simulink library "fordypningsprosjekt"  (Simulink 7.1)
values from neighbouring files (symbols this model uses):
  noise = variance.*randn(6,1)    [camsim3.m]
undefined symbols (not defined in the file or in its folder): bottom_signature, C_calc, ekf2, kalmanfilter, kalmanfilter2
libraries: marine_gnc x5, simulink_extras x3, vrlib x2, simulink x1
(part 1 of 2)
settings Model: Creator=anderga  LastModifiedBy=anderga

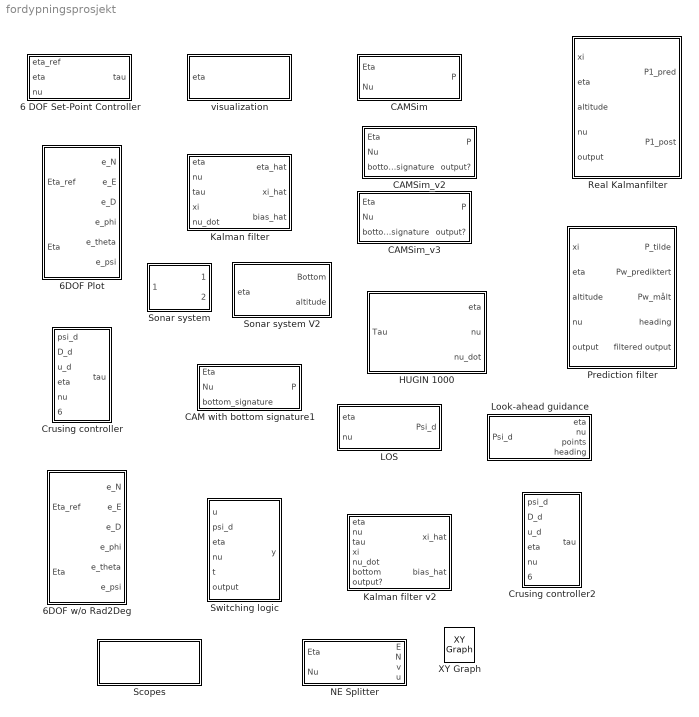
== system fordypningsprosjekt ==
  6 DOF Set-Point Controller : Subsystem  mask(6 DOF Set-point controller){Kp=diag([230 300 1000]), Ki=diag([2 5 0]), Kd=diag([750 700 0]), depthPID=[50, 1, 0], rollPID=[0, 0, 0], pitchPID=[500, 2, 50], sat=1000.*[1, 1, 1, 1, 1, 1]}
      mask prompts: Kp "NE-yaw PID Kp"; Ki "NE-yaw PID Ki"; Kd "NE-yaw PID Kd"; depthPID "Depth PID ([Kp, Ki, Kd])"; rollPID "Roll PID ([Kp, Ki, Kd]) Usually zero, no control moments in roll"; pitchPID "Pitch PID ([Kp, Ki, Kd])"; sat "Forces and Moments Saturation[X, Y, Z, K, M, N]"
      mask init:
      | if isempty(Kp)
      |     Kp = diag([230 300 1000]);
      | end
      | if isempty(Kd)
      |     Kd = diag([750 700 0]);
      | end
      | if isempty(Ki)
      |     Ki = diag([2 5 0]);
      | end
      | if isempty(depthPID)
      |     depthPID = [50, 1, 0];
      | end
      | if isempty(rollPID)
      |     rollPID = [0 0 0];
      | end
      | if isempty(pitchPID)
      |     pitchPID = [500, 2, 50];
      | end
  6DOF Plot : Subsystem
      mask Type: 6 DOF plot reference versus eta
  6DOF w/o Rad2Deg : Subsystem  AncestorBlock=fordypningsprosjekt/6DOF Plot
      mask Type: 6 DOF plot reference versus eta
  CAM with bottom signature1 : Subsystem  AncestorBlock=fordypningsprosjekt/CAM with bottom signature  mask(CAMSim){Noise=off, Variance=0}
      mask prompts: Noise "Noise?"; Variance "Variance noise"
      mask help: Outputs 3 points along the pipeline in the field of view
  CAMSim : Subsystem  mask(CAMSim){bottom=10}
      mask prompts: bottom "Sea Bottom [m]"
      mask help: Outputs 3 points along the pipeline in the field of view
  CAMSim_v2 : Subsystem  AncestorBlock=fordypningsprosjekt/CAMSim
  CAMSim_v3 : Subsystem  AncestorBlock=fordypningsprosjekt/CAMSim_v2  mask{noise=off, variance=0}
      mask prompts: noise "Noise On?"; variance "Noise Variance"
  Crusing controller : Subsystem  AncestorBlock=fordypningsprosjekt/Crusing controller  mask{Kp_u=10, Ki_u=3, Kp_c=100, Kd_c=50, Kp_d=50, Kp2_d=20, Kd_d=20}
      mask prompts: Kp_u "Kp Speed controller"; Ki_u "Ki Speed Controller"; Kp_c "Kp Course Controller"; Kd_c "Kd Course Controller"; Kp_d "Kp1 Depth Controller"; Kp2_d "Kp2 Depth controller"; Kd_d "Kd Depth Controller"
  Crusing controller2 : Subsystem  AncestorBlock=fordypningsprosjekt/Crusing controller2  mask{Kp_u=10, Ki_u=3, K_hp=50, K_hd=20, K_hi=2, T=0.01, K_dp=10, K_di=0.05, K_dd=50}
      mask prompts: Kp_u "Kp Speed controller"; Ki_u "Ki Speed Controller"; K_hp "Kp Course Controller"; K_hd "Kd Course Controller"; K_hi "Ki Course Controller"; T "T Reference feed forward"; K_dp "Kp Depth Controller"; K_di "Ki Depth controller"; K_dd "Kd Depth Controller"
  HUGIN 1000 : Subsystem  AncestorBlock=fordypningsprosjekt/HUGIN 1000  mask(HUGIN 1000 AUV){eta_0=[0 0 0 0 0 0], nu_0=[0 0 0 0 0 0], c_on_off=off, beta_c=-45, V_c=0.3}
      mask prompts: eta_0 "Initial Position [x y z phi theta psi]"; nu_0 "Initial speed [u v w p q r]"; c_on_off "Current on"; beta_c "Current heading(deg)"; V_c "Current Velocity"
      mask help:
      | The hydrodynamic model of Kongsberg Maritimes
      | AUV type HUGIN 1000.
      |
      | Implemented using
      |
      | eta_dot = J(eta)*nu
      | M*nu_dot + C(nu)*nu + D(nu)*nu + g(eta) = tau
      |
      | and the MMS toolbox from www.marinecybernetics.org
      mask init:
      | m = 1380;
      | xg = 0;
      | yg = 0;
      | zg = 0.0328;
      | Ix = 86.53;
      | Iy = 1247;
      | Iz = 1247;
      | 
      | Xu = -85.57;
      | Yv = -1092.9;
      | Yr = -84.1448;
      | Zw = -1092.9;
      | Zq = 84.1448;
      | Mq = -795.1686;
      | Nr = -795.1686;
      |     
      | M = [m-Xu   0       0       0       m*zg    -m*yg;
      |      0      m-Yv    0       -m*zg   0       m*xg-Yr;
      |      0      0       m-Zw    m*yg    -m*xg-Zq 0;
      |      0      -m*zg   m*yg    Ix      0        0;
      |      m*zg   0       -m*xg-Zq 0      Iy-Mq    0;
      |      -m*yg  m*xg-Yr 0       0       0       Iz-Nr];
  Kalman filter : Subsystem
  Kalman filter v2 : Subsystem  AncestorBlock=fordypningsprosjekt/Kalman filter
  LOS : Subsystem
  Look-ahead guidance : Subsystem  Orientation=left  AncestorBlock=fordypningsprosjekt/LOS
  NE Splitter : Subsystem
  Prediction filter : Subsystem
  Real Kalmanfilter : Subsystem
  Scopes : Subsystem
  Sonar system : Subsystem  mask{amplitude=4, bias=50}
      mask prompts: amplitude "Amplitude of bottom signature"; bias "Depth"
  Sonar system V2 : Subsystem  mask{sea_bottom=50}
      mask prompts: sea_bottom "Seabottom [m]"
      mask init:
      | load('bottom_signature')
  Switching logic : Stateflow chart
  XY Graph : simulink/Sinks/XY Graph  SystemSampleTime=-1  xmin=-1000  xmax=1000  ymin=-1000  ymax=1000  st=-1
  visualization : Subsystem

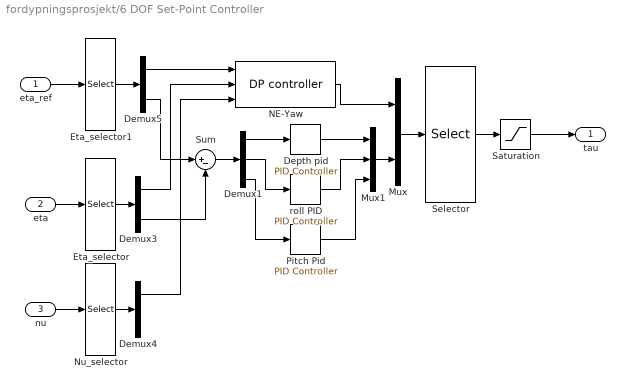
== system fordypningsprosjekt/6 DOF Set-Point Controller ==
  eta_ref : Inport  OutDataType=sfix(16)  OutScaling=2^0
  eta : Inport  Port=2  OutDataType=sfix(16)  OutScaling=2^0
  nu : Inport  Port=3  OutDataType=sfix(16)  OutScaling=2^0
  Demux1 : Demux  Outputs=3
  Demux3 : Demux  Outputs=2
  Demux4 : Demux  Outputs=2
  Demux5 : Demux  Outputs=2
  Depth pid : simulink_extras/Additional Linear/PID Controller  SystemSampleTime=-1  P=depthPID(1)  I=depthPID(2)  D=depthPID(3)
  Eta_selector : Selector  InputPortWidth=6  IndexOptions=Index vector (dialog)  Indices=[1 2 6 3 4 5]  OutputSizes=1
  Eta_selector1 : Selector  InputPortWidth=6  IndexOptions=Index vector (dialog)  Indices=[1 2 6 3 4 5]  OutputSizes=1
  Mux : Mux  Inputs=2
  Mux1 : Mux  Inputs=3
  NE-Yaw : marine_gnc/Control/Dynamic  Positioning /DP controller  SystemSampleTime=-1  Kp=diag([230 300 1000])  Kd=diag([750 700 0])  Ki=diag([2 5 0])
  Nu_selector : Selector  InputPortWidth=6  IndexOptions=Index vector (dialog)  Indices=[1 2 6 3 4 5]  OutputSizes=1
  Pitch Pid : simulink_extras/Additional Linear/PID Controller  SystemSampleTime=-1  P=pitchPID(1)  I=pitchPID(2)  D=pitchPID(3)
  Saturation : Saturate  UpperLimit=sat  LowerLimit=-sat  OutDataType=sfix(16)  OutScaling=2^0
  Selector : Selector  InputPortWidth=6  IndexOptions=Index vector (dialog)  Indices=[1 2 4 5 6 3]  OutputSizes=1
  Sum : Sum  Inputs=|+-  OutDataType=sfix(16)  OutScaling=2^0
  roll PID : simulink_extras/Additional Linear/PID Controller  SystemSampleTime=-1  P=rollPID(1)  I=rollPID(2)  D=rollPID(3)
  tau : Outport  OutDataType=sfix(16)  OutScaling=2^0
  wires:
  Pitch Pid/1 -> Mux1/3
  Demux1/3 -> Pitch Pid/1
  roll PID/1 -> Mux1/2
  Demux1/2 -> roll PID/1
  Depth pid/1 -> Mux1/1
  Demux1/1 -> Depth pid/1
  Sum/1 -> Demux1/1
  Demux3/2 -> Sum/2
  Eta_selector1/1 -> Demux5/1
  Demux5/1 -> NE-Yaw/1
  Demux5/2 -> Sum/1
  eta_ref/1 -> Eta_selector1/1
  Saturation/1 -> tau/1
  Selector/1 -> Saturation/1
  nu/1 -> Nu_selector/1
  eta/1 -> Eta_selector/1
  Demux4/1 -> NE-Yaw/3
  Nu_selector/1 -> Demux4/1
  Demux3/1 -> NE-Yaw/2
  Eta_selector/1 -> Demux3/1
  Mux1/1 -> Mux/2
  Mux/1 -> Selector/1
  NE-Yaw/1 -> Mux/1

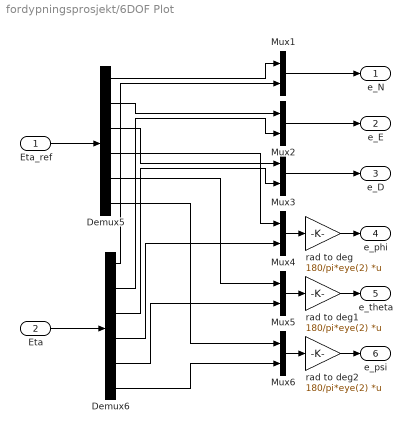
== system fordypningsprosjekt/6DOF Plot ==
  Eta_ref : Inport  OutDataType=sfix(16)  OutScaling=2^0
  Eta : Inport  Port=2  OutDataType=sfix(16)  OutScaling=2^0
  Demux5 : Demux  Outputs=6
  Demux6 : Demux  Outputs=6
  Mux{1..6} (6 alike) : Mux  Inputs=2
  rad to deg : Gain  Gain=180/pi*eye(2)  Multiplication=Matrix(K*u)  ParameterDataType=sfix(16)  ParameterScaling=2^0  OutDataType=sfix(16)  OutScaling=2^0
  rad to deg1 : Gain  Gain=180/pi*eye(2)  Multiplication=Matrix(K*u)  ParameterDataType=sfix(16)  ParameterScaling=2^0  OutDataType=sfix(16)  OutScaling=2^0
  rad to deg2 : Gain  Gain=180/pi*eye(2)  Multiplication=Matrix(K*u)  ParameterDataType=sfix(16)  ParameterScaling=2^0  OutDataType=sfix(16)  OutScaling=2^0
  e_N : Outport  OutDataType=sfix(16)  OutScaling=2^0
  e_E : Outport  Port=2  OutDataType=sfix(16)  OutScaling=2^0
  e_D : Outport  Port=3  OutDataType=sfix(16)  OutScaling=2^0
  e_phi : Outport  Port=4  OutDataType=sfix(16)  OutScaling=2^0
  e_theta : Outport  Port=5  OutDataType=sfix(16)  OutScaling=2^0
  e_psi : Outport  Port=6  OutDataType=sfix(16)  OutScaling=2^0
  wires:
  rad to deg2/1 -> e_psi/1
  rad to deg1/1 -> e_theta/1
  rad to deg/1 -> e_phi/1
  Eta_ref/1 -> Demux5/1
  Demux5/6 -> Mux6/1
  Demux6/6 -> Mux6/2
  Demux6/5 -> Mux5/2
  Demux5/5 -> Mux5/1
  Demux6/4 -> Mux4/2
  Demux5/4 -> Mux4/1
  Mux6/1 -> rad to deg2/1
  Mux5/1 -> rad to deg1/1
  Mux4/1 -> rad to deg/1
  Mux3/1 -> e_D/1
  Mux2/1 -> e_E/1
  Mux1/1 -> e_N/1
  Eta/1 -> Demux6/1
  Demux6/3 -> Mux3/2
  Demux6/2 -> Mux2/2
  Demux5/3 -> Mux3/1
  Demux5/2 -> Mux2/1
  Demux6/1 -> Mux1/2
  Demux5/1 -> Mux1/1

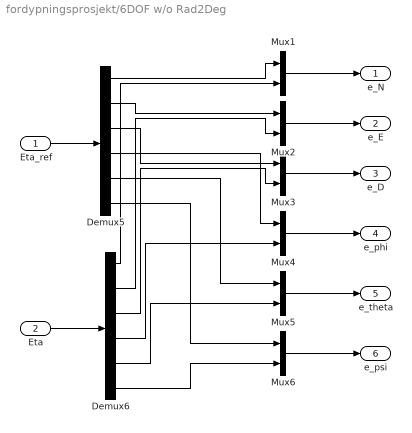
== system fordypningsprosjekt/6DOF w/o Rad2Deg ==
  Eta_ref : Inport  OutDataType=sfix(16)  OutScaling=2^0
  Eta : Inport  Port=2  OutDataType=sfix(16)  OutScaling=2^0
  Demux5 : Demux  Outputs=6
  Demux6 : Demux  Outputs=6
  Mux{1..6} (6 alike) : Mux  Inputs=2
  e_N : Outport  OutDataType=sfix(16)  OutScaling=2^0
  e_E : Outport  Port=2  OutDataType=sfix(16)  OutScaling=2^0
  e_D : Outport  Port=3  OutDataType=sfix(16)  OutScaling=2^0
  e_phi : Outport  Port=4  OutDataType=sfix(16)  OutScaling=2^0
  e_theta : Outport  Port=5  OutDataType=sfix(16)  OutScaling=2^0
  e_psi : Outport  Port=6  OutDataType=sfix(16)  OutScaling=2^0
  wires:
  Eta_ref/1 -> Demux5/1
  Demux5/6 -> Mux6/1
  Demux6/6 -> Mux6/2
  Demux6/5 -> Mux5/2
  Demux5/5 -> Mux5/1
  Demux6/4 -> Mux4/2
  Demux5/4 -> Mux4/1
  Mux6/1 -> e_psi/1
  Mux5/1 -> e_theta/1
  Mux4/1 -> e_phi/1
  Mux3/1 -> e_D/1
  Mux2/1 -> e_E/1
  Mux1/1 -> e_N/1
  Eta/1 -> Demux6/1
  Demux6/3 -> Mux3/2
  Demux6/2 -> Mux2/2
  Demux5/3 -> Mux3/1
  Demux5/2 -> Mux2/1
  Demux6/1 -> Mux1/2
  Demux5/1 -> Mux1/1

== system fordypningsprosjekt/CAM with bottom signature1 ==
  Eta : Inport  OutDataType=sfix(16)  OutScaling=2^0
  Nu : Inport  Port=2  OutDataType=sfix(16)  OutScaling=2^0
  bottom_signature : Inport  Port=3  OutDataType=sfix(16)  OutScaling=2^0
  Clock : Clock
  Constant : Constant  Value=[noise; Variance]  OutDataType=sfix(16)  OutScaling=2^0
  Demux : Demux  Outputs=2
  Euler angles to rotation matrix : Subsystem  AncestorBlock=marine_gnc/Models/ Kinematics/Euler angles to rotation matrix
      mask Type: Euler2R
      mask Description:
      | Determine the 3-by-3 rotation matrix from the Euler angles (roll, pitch, yaw) using the zyx convention.
      | 
      | Output is a 9x1 vector
      mask Display:
      | port_label('input',1,'theta')
      | port_label('output',1,'R')
  Euler angles to attitude transformation matrix : Subsystem  AncestorBlock=marine_gnc/Models/ Kinematics/Euler angles to attitude transformation matrix
      mask Type: Euler2T
      mask Description: Determine the 3-by-3 attitude transformation matrix  from the Euler angles (roll, pitch, yaw).
      mask Display:
      | port_label('input',1,'theta')
      | port_label('output',1,'T')
  MATLAB Fcn : MATLABFcn  MATLABFcn=camsim2  OutputDimensions=6
  Mux : Mux  Inputs=7
  Terminator : Terminator
  P : Outport  OutDataType=sfix(16)  OutScaling=2^0
  wires:
  Constant/1 -> Mux/7
  Clock/1 -> Mux/6
  Euler angles to attitude transformation matrix/1(T) -> Mux/5
  Euler angles to rotation matrix/1(Rzyx) -> Mux/4
  Demux/1 -> Terminator/1
  Demux/2 -> Euler angles to rotation matrix/1(theta), Euler angles to attitude transformation matrix/1(theta)
  MATLAB Fcn/1 -> P/1
  Mux/1 -> MATLAB Fcn/1
  bottom_signature/1 -> Mux/3
  Nu/1 -> Mux/2
  Eta/1 -> Demux/1, Mux/1

== system fordypningsprosjekt/CAMSim ==
  Eta : Inport  OutDataType=sfix(16)  OutScaling=2^0
  Nu : Inport  Port=2  OutDataType=sfix(16)  OutScaling=2^0
  Clock : Clock
  Demux : Demux  Outputs=2
  Euler angles to rotation matrix : Subsystem  AncestorBlock=marine_gnc/Models/ Kinematics/Euler angles to rotation matrix
      mask Type: Euler2R
      mask Description:
      | Determine the 3-by-3 rotation matrix from the Euler angles (roll, pitch, yaw) using the zyx convention.
      | 
      | Output is a 9x1 vector
      mask Display:
      | port_label('input',1,'theta')
      | port_label('output',1,'R')
  Euler angles to attitude transformation matrix : Subsystem  AncestorBlock=marine_gnc/Models/ Kinematics/Euler angles to attitude transformation matrix
      mask Type: Euler2T
      mask Description: Determine the 3-by-3 attitude transformation matrix  from the Euler angles (roll, pitch, yaw).
      mask Display:
      | port_label('input',1,'theta')
      | port_label('output',1,'T')
  MATLAB Fcn : MATLABFcn  MATLABFcn=camsim2  OutputDimensions=6
  Mux : Mux  Inputs=6
  Terminator : Terminator
  bottom : Constant  Value=bottom  OutDataType=sfix(16)  OutScaling=2^0
  P : Outport  OutDataType=sfix(16)  OutScaling=2^0
  wires:
  Clock/1 -> Mux/6
  Euler angles to attitude transformation matrix/1(T) -> Mux/5
  Euler angles to rotation matrix/1(Rzyx) -> Mux/4
  Demux/1 -> Terminator/1
  Demux/2 -> Euler angles to rotation matrix/1(theta), Euler angles to attitude transformation matrix/1(theta)
  MATLAB Fcn/1 -> P/1
  Mux/1 -> MATLAB Fcn/1
  bottom/1 -> Mux/3
  Nu/1 -> Mux/2
  Eta/1 -> Demux/1, Mux/1

== system fordypningsprosjekt/CAMSim_v2 ==
  Eta : Inport  OutDataType=sfix(16)  OutScaling=2^0
  Nu : Inport  Port=2  OutDataType=sfix(16)  OutScaling=2^0
  bottom_signature : Inport  Port=3  OutDataType=sfix(16)  OutScaling=2^0
  Clock : Clock
  Demux : Demux  Outputs=2
  Euler angles to rotation matrix : Subsystem  AncestorBlock=marine_gnc/Models/ Kinematics/Euler angles to rotation matrix
      mask Type: Euler2R
      mask Description:
      | Determine the 3-by-3 rotation matrix from the Euler angles (roll, pitch, yaw) using the zyx convention.
      | 
      | Output is a 9x1 vector
      mask Display:
      | port_label('input',1,'theta')
      | port_label('output',1,'R')
  Euler angles to attitude transformation matrix : Subsystem  AncestorBlock=marine_gnc/Models/ Kinematics/Euler angles to attitude transformation matrix
      mask Type: Euler2T
      mask Description: Determine the 3-by-3 attitude transformation matrix  from the Euler angles (roll, pitch, yaw).
      mask Display:
      | port_label('input',1,'theta')
      | port_label('output',1,'T')
  MATLAB Fcn : MATLABFcn  MATLABFcn=camsim3  OutputDimensions=7
  Mux : Mux  Inputs=6
  Selector : Selector  InputPortWidth=7  IndexOptions=Index vector (dialog)  Indices=[1 2 3 4 5 6]  OutputSizes=1
  Selector1 : Selector  InputPortWidth=7  IndexOptions=Index vector (dialog)  Indices=[7]  OutputSizes=1
  Terminator : Terminator
  P : Outport  OutDataType=sfix(16)  OutScaling=2^0
  output? : Outport  Port=2  OutDataType=sfix(16)  OutScaling=2^0
  wires:
  Selector1/1 -> output?/1
  Selector/1 -> P/1
  MATLAB Fcn/1 -> Selector/1, Selector1/1
  Clock/1 -> Mux/6
  Euler angles to attitude transformation matrix/1(T) -> Mux/5
  Euler angles to rotation matrix/1(Rzyx) -> Mux/4
  Demux/1 -> Terminator/1
  Demux/2 -> Euler angles to rotation matrix/1(theta), Euler angles to attitude transformation matrix/1(theta)
  Mux/1 -> MATLAB Fcn/1
  bottom_signature/1 -> Mux/3
  Nu/1 -> Mux/2
  Eta/1 -> Demux/1, Mux/1

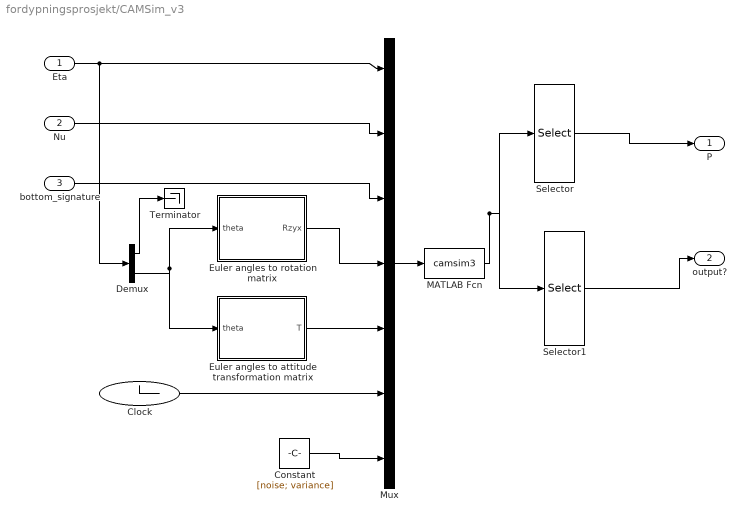
== system fordypningsprosjekt/CAMSim_v3 ==
  Eta : Inport  OutDataType=sfix(16)  OutScaling=2^0
  Nu : Inport  Port=2  OutDataType=sfix(16)  OutScaling=2^0
  bottom_signature : Inport  Port=3  OutDataType=sfix(16)  OutScaling=2^0
  Clock : Clock
  Constant : Constant  Value=[noise; variance]  OutDataType=sfix(16)  OutScaling=2^0
  Demux : Demux  Outputs=2
  Euler angles to rotation matrix : Subsystem  AncestorBlock=marine_gnc/Models/ Kinematics/Euler angles to rotation matrix
      mask Type: Euler2R
      mask Description:
      | Determine the 3-by-3 rotation matrix from the Euler angles (roll, pitch, yaw) using the zyx convention.
      | 
      | Output is a 9x1 vector
      mask Display:
      | port_label('input',1,'theta')
      | port_label('output',1,'R')
  Euler angles to attitude transformation matrix : Subsystem  AncestorBlock=marine_gnc/Models/ Kinematics/Euler angles to attitude transformation matrix
      mask Type: Euler2T
      mask Description: Determine the 3-by-3 attitude transformation matrix  from the Euler angles (roll, pitch, yaw).
      mask Display:
      | port_label('input',1,'theta')
      | port_label('output',1,'T')
  MATLAB Fcn : MATLABFcn  MATLABFcn=camsim3  OutputDimensions=7
  Mux : Mux  Inputs=7
  Selector : Selector  InputPortWidth=7  IndexOptions=Index vector (dialog)  Indices=[1 2 3 4 5 6]  OutputSizes=1
  Selector1 : Selector  InputPortWidth=7  IndexOptions=Index vector (dialog)  Indices=[7]  OutputSizes=1
  Terminator : Terminator
  P : Outport  OutDataType=sfix(16)  OutScaling=2^0
  output? : Outport  Port=2  OutDataType=sfix(16)  OutScaling=2^0
  wires:
  Constant/1 -> Mux/7
  Selector1/1 -> output?/1
  Selector/1 -> P/1
  MATLAB Fcn/1 -> Selector/1, Selector1/1
  Clock/1 -> Mux/6
  Euler angles to attitude transformation matrix/1(T) -> Mux/5
  Euler angles to rotation matrix/1(Rzyx) -> Mux/4
  Demux/1 -> Terminator/1
  Demux/2 -> Euler angles to rotation matrix/1(theta), Euler angles to attitude transformation matrix/1(theta)
  Mux/1 -> MATLAB Fcn/1
  bottom_signature/1 -> Mux/3
  Nu/1 -> Mux/2
  Eta/1 -> Demux/1, Mux/1

== system fordypningsprosjekt/Crusing controller ==
  psi_d : Inport  OutDataType=sfix(16)  OutScaling=2^0
  D_d : Inport  Port=2  OutDataType=sfix(16)  OutScaling=2^0
  u_d : Inport  Port=3  OutDataType=sfix(16)  OutScaling=2^0
  eta : Inport  Port=4  OutDataType=sfix(16)  OutScaling=2^0
  nu : Inport  Port=5  OutDataType=sfix(16)  OutScaling=2^0
  nu_dot : Inport  Port=6  OutDataType=sfix(16)  OutScaling=2^0
  Demux : Demux  Outputs=6
  Demux1 : Demux  Outputs=6
  Mux : Mux  Inputs=6
  bottom : Constant  Value=0  OutDataType=sfix(16)  OutScaling=2^0
  course control : Subsystem
  depth : Subsystem
  speed : Subsystem
  tau : Outport  OutDataType=sfix(16)  OutScaling=2^0
  wires:
  bottom/1 -> Mux/4
  depth/2(tau_5) -> Mux/5
  depth/1(tau_3) -> Mux/3
  Demux1/5 -> depth/4(theta)
  Demux/5 -> depth/3(q)
  Demux1/3 -> depth/1(D)
  D_d/1 -> depth/2(D_d)
  course control/2(tau_6) -> Mux/6
  course control/1(tau_2) -> Mux/2
  Mux/1 -> tau/1
  speed/1(Out1) -> Mux/1
  Demux/6 -> course control/3(r)
  psi_d/1 -> course control/2(psi_d)
  Demux1/6 -> course control/1(psi)
  eta/1 -> Demux1/1
  u_d/1 -> speed/2(u_d)
  Demux/1 -> speed/1(u)
  nu/1 -> Demux/1

== system fordypningsprosjekt/Crusing controller2 ==
  psi_d : Inport  OutDataType=sfix(16)  OutScaling=2^0
  D_d : Inport  Port=2  OutDataType=sfix(16)  OutScaling=2^0
  u_d : Inport  Port=3  OutDataType=sfix(16)  OutScaling=2^0
  eta : Inport  Port=4  OutDataType=sfix(16)  OutScaling=2^0
  nu : Inport  Port=5  OutDataType=sfix(16)  OutScaling=2^0
  nu_dot : Inport  Port=6  OutDataType=sfix(16)  OutScaling=2^0
  Demux : Demux  Outputs=6
  Demux1 : Demux  Outputs=6
  Mux : Mux  Inputs=6
  bottom : Constant  Value=0  OutDataType=sfix(16)  OutScaling=2^0
  course control : Subsystem
  depth : Subsystem
  speed : Subsystem
  tau : Outport  OutDataType=sfix(16)  OutScaling=2^0
  wires:
  Demux/5 -> depth/4(q)
  Demux1/5 -> depth/3(theta)
  nu/1 -> Demux/1
  Demux/1 -> speed/1(u)
  u_d/1 -> speed/2(u_d)
  eta/1 -> Demux1/1
  Demux1/6 -> course control/1(psi)
  psi_d/1 -> course control/3(psi_d)
  Demux/6 -> course control/2(r)
  speed/1(Out1) -> Mux/1
  Mux/1 -> tau/1
  course control/1(tau_6) -> Mux/6
  D_d/1 -> depth/2(D_d)
  Demux1/3 -> depth/1(D)
  depth/1(tau_5) -> Mux/5
  bottom/1 -> Mux/4, Mux/3, Mux/2

== system fordypningsprosjekt/HUGIN 1000 ==
  Tau : Inport  OutDataType=sfix(16)  OutScaling=2^0
  6 DOF Eqs. of motion : Subsystem  AncestorBlock=marine_gnc/Models/ Kinetics /6 DOF Eqs. of motion  mask(Equations of motion){nu0=nu_0, eta0=eta_0}
      mask prompts: nu0 "Initial velocities (u,v,w,p,q,r)"; eta0 "Initial position/attitude (x,y,z,phi,theta,psi)"
      mask help:
      | 6 DOF equations of motion (surge, sway, heave, roll, pitch and yaw)
      |
      |    eta_dot = J(eta)*nu
      |    (M_RB+M_A)*nu_dot  =  tau
      |
      | where nu = [u,v,w,p,q,r]'  and eta = [x,y,z,phi,theta,psi]'
      |
      | T. I. Fossen (2002). Marine Control Systems: Guidance, Navigation and Control of Ships, Rigs and Underwater Vehicles, Marine Cybernetics AS, ISBN 82-92356-00-2
      |
      | Modified by Anders Garmo (2008)
  C(nu)*nu : Scope
      settings: TimeRange=100  YMin=-0.1  YMax=1.2  SaveName=ScopeData5
  D(nu)*nu : Scope
      settings: TimeRange=100  YMin=-10  YMax=100  SaveName=ScopeData8
  Mass/Inertia matrix : Constant  Value=M  OutDataType=sfix(16)  OutScaling=2^0
  Sum : Sum  Inputs=|+---  OutDataType=sfix(16)  OutScaling=2^0
  coriolis  forces : Subsystem  Orientation=left
      mask init:
      | W = 1380*9.81;
      | 
      | zg = 0.0328;
  damping : Subsystem  Orientation=left
      mask init:
      | Xu = -19.1881;
      | Yv = -931.9715;
      | Yr = 1915.8;
      | Zw = -931.9715;
      | Zq = -1915.8;
      | Kp = -1000;
      | Mw = 1760.7;
      | Mq = -8386.3;
      | Nv = -1760.7;
      | Nr = -8386.3;
      | 
      | Xuu = -3.8938;
      | 
      | D = [Xu 0 0 0 0 0;
      |       0 Yv 0 0 0 Yr;
      |       0 0 Zw 0 Zq 0;
      |       0 0 0 Kp 0 0;
      |       0 0 Mw 0 Mq 0;
      |       0 Nv 0 0 0 Nr];
  g(eta) : Scope
      settings: TimeRange=100  YMin=0  YMax=100  SaveName=ScopeData7
  restoring forces : Subsystem  Orientation=left
      mask init:
      | W = 1380*9.81;
      | 
      | zg = 0.0328;
  eta : Outport  OutDataType=sfix(16)  OutScaling=2^0
  nu : Outport  Port=2  OutDataType=sfix(16)  OutScaling=2^0
  nu_dot : Outport  Port=3  OutDataType=sfix(16)  OutScaling=2^0
  wires:
  6 DOF Eqs. of motion/3(nu_dot) -> nu_dot/1
  damping/1(D(nu)*nu) -> D(nu)*nu/1, Sum/3
  restoring forces/1(g(eta)) -> g(eta)/1, Sum/4
  coriolis  forces/1(C(nu)*nu) -> Sum/2, C(nu)*nu/1
  Tau/1 -> Sum/1
  Sum/1 -> 6 DOF Eqs. of motion/2(tau)
  6 DOF Eqs. of motion/1(eta) -> eta/1, restoring forces/1(eta)
  6 DOF Eqs. of motion/2(nu) -> coriolis  forces/1(nu), damping/1(nu), nu/1
  Mass/Inertia matrix/1 -> 6 DOF Eqs. of motion/1(M)

== system fordypningsprosjekt/Kalman filter ==
  eta : Inport  OutDataType=sfix(16)  OutScaling=2^0
  nu : Inport  Port=2  OutDataType=sfix(16)  OutScaling=2^0
  tau : Inport  Port=3  OutDataType=sfix(16)  OutScaling=2^0
  xi : Inport  Port=4  OutDataType=sfix(16)  OutScaling=2^0
  nu_dot : Inport  Port=5  OutDataType=sfix(16)  OutScaling=2^0
  Demux : Demux  Outputs=3
  Mux : Mux  Inputs=5
  ekf file : MATLABFcn  MATLABFcn=ekf2(u)  OutputDimensions=18
  eta_hat : Outport  OutDataType=sfix(16)  OutScaling=2^0
  xi_hat : Outport  Port=2  OutDataType=sfix(16)  OutScaling=2^0
  bias_hat : Outport  Port=3  OutDataType=sfix(16)  OutScaling=2^0
  wires:
  nu_dot/1 -> Mux/5
  nu/1 -> Mux/4
  tau/1 -> Mux/3
  xi/1 -> Mux/2
  ekf file/1 -> Demux/1
  Mux/1 -> ekf file/1
  Demux/3 -> bias_hat/1
  Demux/2 -> xi_hat/1
  Demux/1 -> eta_hat/1
  eta/1 -> Mux/1

== system fordypningsprosjekt/Kalman filter v2 ==
  eta : Inport  OutDataType=sfix(16)  OutScaling=2^0
  nu : Inport  Port=2  OutDataType=sfix(16)  OutScaling=2^0
  tau : Inport  Port=3  OutDataType=sfix(16)  OutScaling=2^0
  xi : Inport  Port=4  OutDataType=sfix(16)  OutScaling=2^0
  nu_dot : Inport  Port=5  OutDataType=sfix(16)  OutScaling=2^0
  bottom : Inport  Port=6  OutDataType=sfix(16)  OutScaling=2^0
  output? : Inport  Port=7  OutDataType=sfix(16)  OutScaling=2^0
  Demux : Demux  Outputs=2
  Mux : Mux  Inputs=7
  ekf file : MATLABFcn  MATLABFcn=ekf2(u)  OutputDimensions=12
  xi_hat : Outport  OutDataType=sfix(16)  OutScaling=2^0
  bias_hat : Outport  Port=2  OutDataType=sfix(16)  OutScaling=2^0
  wires:
  output?/1 -> Mux/7
  Demux/2 -> bias_hat/1
  Demux/1 -> xi_hat/1
  bottom/1 -> Mux/6
  nu_dot/1 -> Mux/5
  nu/1 -> Mux/4
  tau/1 -> Mux/3
  xi/1 -> Mux/2
  ekf file/1 -> Demux/1
  Mux/1 -> ekf file/1
  eta/1 -> Mux/1

== system fordypningsprosjekt/LOS ==
  eta : Inport  OutDataType=sfix(16)  OutScaling=2^0
  nu : Inport  Port=2  OutDataType=sfix(16)  OutScaling=2^0
  MATLAB Fcn : MATLABFcn  MATLABFcn=los_calc  OutputDimensions=1
  Mux : Mux  Inputs=2
  Psi_d : Outport  OutDataType=sfix(16)  OutScaling=2^0
  wires:
  MATLAB Fcn/1 -> Psi_d/1
  Mux/1 -> MATLAB Fcn/1
  nu/1 -> Mux/2
  eta/1 -> Mux/1

== system fordypningsprosjekt/Look-ahead guidance ==
  eta : Inport  OutDataType=sfix(16)  OutScaling=2^0
  nu : Inport  Port=2  OutDataType=sfix(16)  OutScaling=2^0
  points : Inport  Port=3  OutDataType=sfix(16)  OutScaling=2^0
  heading : Inport  Port=4  OutDataType=sfix(16)  OutScaling=2^0
  Mux : Mux
  lah-guidance : MATLABFcn  MATLABFcn=lah_guidance  OutputDimensions=1
  Psi_d : Outport  OutDataType=sfix(16)  OutScaling=2^0
  wires:
  heading/1 -> Mux/4
  points/1 -> Mux/3
  eta/1 -> Mux/1
  nu/1 -> Mux/2
  Mux/1 -> lah-guidance/1
  lah-guidance/1 -> Psi_d/1

== system fordypningsprosjekt/NE Splitter ==
  Eta : Inport  OutDataType=sfix(16)  OutScaling=2^0
  Nu : Inport  Port=2  OutDataType=sfix(16)  OutScaling=2^0
  Demux : Demux  Outputs=2
  Demux1 : Demux  Outputs=2
  Selector1 : Selector  InputPortWidth=6  IndexOptions=Index vector (dialog)  Indices=[1 2]  OutputSizes=1
  Selector2 : Selector  InputPortWidth=6  IndexOptions=Index vector (dialog)  Indices=[1 2]  OutputSizes=1
  E : Outport  OutDataType=sfix(16)  OutScaling=2^0
  N : Outport  Port=2  OutDataType=sfix(16)  OutScaling=2^0
  v : Outport  Port=3  OutDataType=sfix(16)  OutScaling=2^0
  u : Outport  Port=4  OutDataType=sfix(16)  OutScaling=2^0
  wires:
  Eta/1 -> Selector2/1
  Nu/1 -> Selector1/1
  Selector2/1 -> Demux/1
  Demux/1 -> N/1
  Demux/2 -> E/1
  Selector1/1 -> Demux1/1
  Demux1/1 -> u/1
  Demux1/2 -> v/1

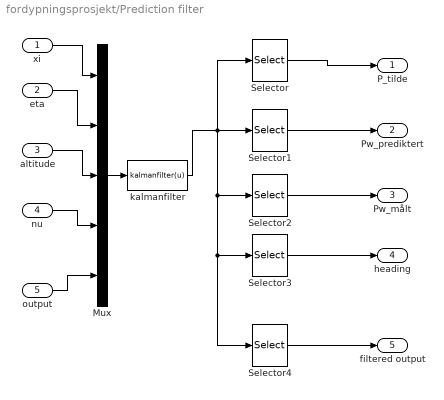
== system fordypningsprosjekt/Prediction filter ==
  xi : Inport  OutDataType=sfix(16)  OutScaling=2^0
  eta : Inport  Port=2  OutDataType=sfix(16)  OutScaling=2^0
  altitude : Inport  Port=3  OutDataType=sfix(16)  OutScaling=2^0
  nu : Inport  Port=4  OutDataType=sfix(16)  OutScaling=2^0
  output : Inport  Port=5  OutDataType=sfix(16)  OutScaling=2^0
  Mux : Mux  Inputs=5
  Selector : Selector  InputPortWidth=29  IndexOptions=Index vector (dialog)  Indices=[1:9]  OutputSizes=1
  Selector1 : Selector  InputPortWidth=29  IndexOptions=Index vector (dialog)  Indices=[10:12]  OutputSizes=1
  Selector2 : Selector  InputPortWidth=29  IndexOptions=Index vector (dialog)  Indices=[13:21]  OutputSizes=1
  Selector3 : Selector  InputPortWidth=29  IndexOptions=Index vector (dialog)  Indices=22:23  OutputSizes=1
  Selector4 : Selector  InputPortWidth=29  IndexOptions=Index vector (dialog)  Indices=24:29  OutputSizes=1
  kalmanfilter : MATLABFcn  MATLABFcn=kalmanfilter(u)  OutputDimensions=29
  P_tilde : Outport  OutDataType=sfix(16)  OutScaling=2^0
  Pw_prediktert : Outport  Port=2  OutDataType=sfix(16)  OutScaling=2^0
  Pw_målt : Outport  Port=3  OutDataType=sfix(16)  OutScaling=2^0
  heading : Outport  Port=4  OutDataType=sfix(16)  OutScaling=2^0
  filtered output : Outport  Port=5  OutDataType=sfix(16)  OutScaling=2^0
  wires:
  output/1 -> Mux/5
  Selector4/1 -> filtered output/1
  Selector3/1 -> heading/1
  Selector2/1 -> Pw_målt/1
  Selector1/1 -> Pw_prediktert/1
  kalmanfilter/1 -> Selector4/1, Selector3/1, Selector2/1, Selector1/1, Selector/1
  Selector/1 -> P_tilde/1
  Mux/1 -> kalmanfilter/1
  nu/1 -> Mux/4
  altitude/1 -> Mux/3
  eta/1 -> Mux/2
  xi/1 -> Mux/1

== system fordypningsprosjekt/Real Kalmanfilter ==
  xi : Inport  OutDataType=sfix(16)  OutScaling=2^0
  eta : Inport  Port=2  OutDataType=sfix(16)  OutScaling=2^0
  altitude : Inport  Port=3  OutDataType=sfix(16)  OutScaling=2^0
  nu : Inport  Port=4  OutDataType=sfix(16)  OutScaling=2^0
  output : Inport  Port=5  OutDataType=sfix(16)  OutScaling=2^0
  Mux : Mux  Inputs=5
  Selector : Selector  InputPortWidth=6  IndexOptions=Index vector (dialog)  Indices=[1:3]  OutputSizes=1
  Selector1 : Selector  InputPortWidth=6  IndexOptions=Index vector (dialog)  Indices=4:6  OutputSizes=1
  kalmanfilter : MATLABFcn  MATLABFcn=kalmanfilter2(u)  OutputDimensions=6
  P1_pred : Outport  OutDataType=sfix(16)  OutScaling=2^0
  P1_post : Outport  Port=2  OutDataType=sfix(16)  OutScaling=2^0
  wires:
  Selector1/1 -> P1_post/1
  Selector/1 -> P1_pred/1
  kalmanfilter/1 -> Selector1/1, Selector/1
  xi/1 -> Mux/1
  eta/1 -> Mux/2
  altitude/1 -> Mux/3
  nu/1 -> Mux/4
  Mux/1 -> kalmanfilter/1
  output/1 -> Mux/5

== system fordypningsprosjekt/Scopes ==
  Attitude : Scope  NumInputPorts=3
      settings: YMin=-5~-5~-5  YMax=5~5~5  SaveName=Attitiude
  Sonar : Scope  NumInputPorts=2
      settings: YMin=-5~-5  YMax=5~5  SaveName=Sonar_data
  Translation : Scope  NumInputPorts=3
      settings: YMin=-5~-5~-5  YMax=5~5~5  SaveName=Translation

== system fordypningsprosjekt/Sonar system ==
  depth : Inport  OutDataType=sfix(16)  OutScaling=2^0
  Sum1 : Sum  Inputs=|+-  OutDataType=sfix(16)  OutScaling=2^0
  bottom signature : Sin  Amplitude=amplitude  Bias=bias  Frequency=0.01  SampleTime=0
  Bottom : Outport  OutDataType=sfix(16)  OutScaling=2^0
  altitude : Outport  Port=2  OutDataType=sfix(16)  OutScaling=2^0
  wires:
  Sum1/1 -> altitude/1
  depth/1 -> Sum1/2
  bottom signature/1 -> Sum1/1, Bottom/1

== system fordypningsprosjekt/Sonar system V2 ==
  eta : Inport  OutDataType=sfix(16)  OutScaling=2^0
  Constant : Constant  Value=sea_bottom  OutDataType=sfix(16)  OutScaling=2^0
  Down : Selector  InputPortWidth=6  IndexOptions=Index vector (dialog)  Indices=[3]  OutputSizes=1
  East : Selector  InputPortWidth=6  IndexOptions=Index vector (dialog)  Indices=[2]  OutputSizes=1
  North : Selector  InputPortWidth=6  IndexOptions=Index vector (dialog)  Indices=[1]  OutputSizes=1
  Sea Bottom  signature : Lookup2D  RowIndex=[1:size(bottom_signature)]  ColumnIndex=[1:size(bottom_signature)]  Table=bottom_signature  LookUpMeth=Use Input Nearest  OutDataType=sfix(16)  OutScaling=2^0
  Sum1 : Sum  Inputs=|+-  OutDataType=sfix(16)  OutScaling=2^0
  Sum2 : Sum  Inputs=|++  OutDataType=sfix(16)  OutScaling=2^0
  Bottom : Outport  OutDataType=sfix(16)  OutScaling=2^0
  altitude : Outport  Port=2  OutDataType=sfix(16)  OutScaling=2^0
  wires:
  Constant/1 -> Sum2/2
  Sum2/1 -> Bottom/1, Sum1/1
  Sea Bottom  signature/1 -> Sum2/1
  East/1 -> Sea Bottom  signature/2
  eta/1 -> Down/1, East/1, North/1
  North/1 -> Sea Bottom  signature/1
  Sum1/1 -> altitude/1
  Down/1 -> Sum1/2

== system fordypningsprosjekt/visualization ==
  eta : Inport  OutDataType=sfix(16)  OutScaling=2^0
  -z : Gain  Gain=-1  ParameterDataType=sfix(16)  ParameterScaling=2^0  OutDataType=sfix(16)  OutScaling=2^0
  Constant : Constant  Value=pi/2  OutDataType=sfix(16)  OutScaling=2^0
  Demux2 : Demux  Outputs=2
  Demux3 : Demux  Outputs=3
  Euler angles to inverse rotation matrix : marine_gnc/Models/ Kinematics/Euler angles to inverse rotation matrix  SystemSampleTime=-1
  Mux : Mux  Inputs=3
  Rotation Matrix to VRML Rotation : vrlib/Utilities/Rotation Matrix to VRML Rotation  SystemSampleTime=-1  maxzero=1e-12
  Selector : Selector  InputPortWidth=3  IndexOptions=Index vector (dialog)  Indices=[2 3 1]  OutputSizes=1
  Selector1 : Selector  InputPortWidth=3  IndexOptions=Index vector (dialog)  Indices=[2 1 3]  OutputSizes=1
  Sum : Sum  Inputs=|++  OutDataType=sfix(16)  OutScaling=2^0
  VR Sink : vrlib/VR Sink  SampleTime=-1  ViewEnable=on  RemoteChange=off  RemoteView=off  FieldsWritten=Mounted.orientation.4.1.double#Mounted.position.3.1.double#Hugin1000.rotation.4.1.double#Hugin1000.translation.3.1.double  WorldFileName=M:\tex\svn\3d-modell\hugin.WRL  WorldDescription=HUGIN 1000  AutoView=off  VideoDimensions=[]  FigureProperties="{'Position', 'Name', 'Viewpoint', 'CameraBound', 'CameraDirection', 'CameraPosition', 'CameraUpVector', 'ZoomFactor', 'Antialiasing', 'Headlight', 'Lighting', 'NavPanel', 'StatusBar', 'ToolBar', 'Textures', 'Transparency', 'Wireframe', 'NavZones', 'NavMode', 'NavSpeed', 'Record2DCompressMethod', 'Record2DCompressQuality', 'Record2D', 'Record2DFileName', 'Record2DFPS'; [1.7000000000000000e+001  7.2000000000000000e+001  5.7600000000000000e+002  3.8000000000000000e+002], '', 'Overview', 'on', [0.0000000000000000e+000  0.0000000000000000e+000 -1.0000000000000000e+000], [0.0000000000000000e+000  0.0000000000000000e+000  1.4400000000000000e+002], [0.0000000000000000e+000  1.0000000000000000e+000  0.0000000000000000e+000], [1.0000000000000000e+000], 'off', 'on', 'on', 'halfbar', 'off', 'on', 'on', 'on', 'off', 'off', 'fly', 'normal', 'auto', [7.5000000000000000e+001], 'off', '%f_anim_%n.avi', [1.5000000000000000e+001]}"
  scale gain : Gain  Gain=diag([10 10 10])  Multiplication=Matrix(K*u)  ParameterDataType=sfix(16)  ParameterScaling=2^0  OutDataType=sfix(16)  OutScaling=2^0
  wires:
  scale gain/1 -> VR Sink/4, VR Sink/2
  Rotation Matrix to VRML Rotation/1 -> VR Sink/1, VR Sink/3
  eta/1 -> Demux2/1
  -z/1 -> Mux/3
  Demux3/2 -> Mux/2
  Sum/1 -> Mux/1
  Demux3/1 -> Sum/1
  Constant/1 -> Sum/2
  Demux3/3 -> -z/1
  Mux/1 -> Euler angles to inverse rotation matrix/1
  Selector1/1 -> Demux3/1
  Demux2/2 -> Selector1/1
  Euler angles to inverse rotation matrix/1 -> Rotation Matrix to VRML Rotation/1
  Selector/1 -> scale gain/1
  Demux2/1 -> Selector/1

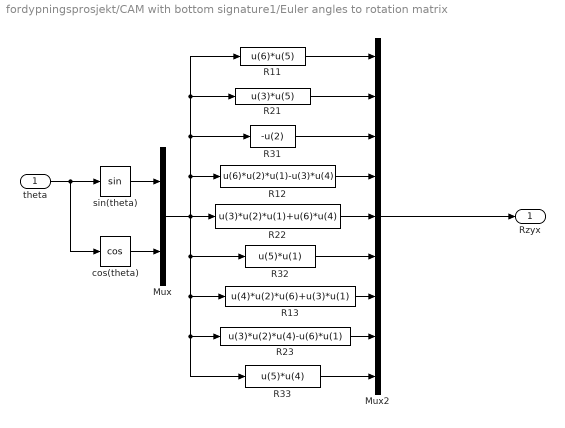
== system fordypningsprosjekt/CAM with bottom signature1/Euler angles to rotation matrix ==
  theta : Inport  OutDataType=sfix(16)  OutScaling=2^0
  Mux : Mux  Inputs=2
  Mux2 : Mux  Inputs=9
  R11 : Fcn  Expr=u(6)*u(5)
  R12 : Fcn  Expr=u(6)*u(2)*u(1)-u(3)*u(4)
  R13 : Fcn  Expr=u(4)*u(2)*u(6)+u(3)*u(1)
  "R21 " : Fcn  Expr=u(3)*u(5)
  R22 : Fcn  Expr=u(3)*u(2)*u(1)+u(6)*u(4)
  R23 : Fcn  Expr=u(3)*u(2)*u(4)-u(6)*u(1)
  "R31 " : Fcn  Expr=-u(2)
  R32 : Fcn  Expr=u(5)*u(1)
  R33 : Fcn  Expr=u(5)*u(4)
  cos(theta) : Trigonometry  Operator=cos
  sin(theta) : Trigonometry
  Rzyx : Outport  OutDataType=sfix(16)  OutScaling=2^0  InitialOutput=0
  wires:
  R11/1 -> Mux2/1
  Mux2/1 -> Rzyx/1
  sin(theta)/1 -> Mux/1
  cos(theta)/1 -> Mux/2
  theta/1 -> sin(theta)/1, cos(theta)/1
  Mux/1 -> R32/1, R13/1, R33/1, R23/1, R22/1, "R31 "/1, R11/1, "R21 "/1, R12/1
  R23/1 -> Mux2/8
  R13/1 -> Mux2/7
  R22/1 -> Mux2/5
  R12/1 -> Mux2/4
  "R31 "/1 -> Mux2/3
  "R21 "/1 -> Mux2/2
  R32/1 -> Mux2/6
  R33/1 -> Mux2/9

== system fordypningsprosjekt/CAM with bottom signature1/Euler angles to attitude transformation matrix ==
  theta : Inport  OutDataType=sfix(16)  OutScaling=2^0
  Constant : Constant  OutDataType=sfix(16)  OutScaling=2^0
  "Constant " : Constant  Value=0  OutDataType=sfix(16)  OutScaling=2^0
  Mux2 : Mux  Inputs=9
  "T21 " : Fcn  Expr=sin(u(1))*tan(u(2))
  T22 : Fcn  Expr=cos(u(1))
  T23 : Fcn  Expr=sin(u(1))/cos(u(2))
  "T31 " : Fcn  Expr=cos(u(1))*tan(u(2))
  T32 : Fcn  Expr=-sin(u(1))
  T33 : Fcn  Expr=cos(u(1))/cos(u(2))
  T : Outport  OutDataType=sfix(16)  OutScaling=2^0  InitialOutput=0
  wires:
  Constant/1 -> Mux2/1
  Mux2/1 -> T/1
  theta/1 -> T23/1, T33/1, T32/1, "T31 "/1, T22/1, "T21 "/1
  T23/1 -> Mux2/6
  T22/1 -> Mux2/5
  T33/1 -> Mux2/9
  "Constant "/1 -> Mux2/2, Mux2/3
  "T21 "/1 -> Mux2/4
  "T31 "/1 -> Mux2/7
  T32/1 -> Mux2/8

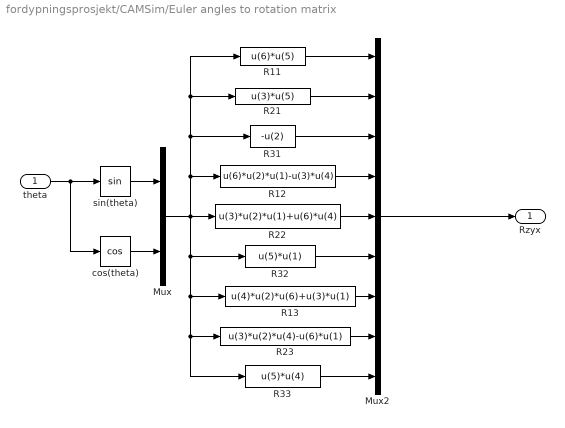
== system fordypningsprosjekt/CAMSim/Euler angles to rotation matrix ==
  theta : Inport  OutDataType=sfix(16)  OutScaling=2^0
  Mux : Mux  Inputs=2
  Mux2 : Mux  Inputs=9
  R11 : Fcn  Expr=u(6)*u(5)
  R12 : Fcn  Expr=u(6)*u(2)*u(1)-u(3)*u(4)
  R13 : Fcn  Expr=u(4)*u(2)*u(6)+u(3)*u(1)
  "R21 " : Fcn  Expr=u(3)*u(5)
  R22 : Fcn  Expr=u(3)*u(2)*u(1)+u(6)*u(4)
  R23 : Fcn  Expr=u(3)*u(2)*u(4)-u(6)*u(1)
  "R31 " : Fcn  Expr=-u(2)
  R32 : Fcn  Expr=u(5)*u(1)
  R33 : Fcn  Expr=u(5)*u(4)
  cos(theta) : Trigonometry  Operator=cos
  sin(theta) : Trigonometry
  Rzyx : Outport  OutDataType=sfix(16)  OutScaling=2^0  InitialOutput=0
  wires:
  R11/1 -> Mux2/1
  Mux2/1 -> Rzyx/1
  sin(theta)/1 -> Mux/1
  cos(theta)/1 -> Mux/2
  theta/1 -> sin(theta)/1, cos(theta)/1
  Mux/1 -> R32/1, R13/1, R33/1, R23/1, R22/1, "R31 "/1, R11/1, "R21 "/1, R12/1
  R23/1 -> Mux2/8
  R13/1 -> Mux2/7
  R22/1 -> Mux2/5
  R12/1 -> Mux2/4
  "R31 "/1 -> Mux2/3
  "R21 "/1 -> Mux2/2
  R32/1 -> Mux2/6
  R33/1 -> Mux2/9

== system fordypningsprosjekt/CAMSim/Euler angles to attitude transformation matrix ==
  theta : Inport  OutDataType=sfix(16)  OutScaling=2^0
  Constant : Constant  OutDataType=sfix(16)  OutScaling=2^0
  "Constant " : Constant  Value=0  OutDataType=sfix(16)  OutScaling=2^0
  Mux2 : Mux  Inputs=9
  "T21 " : Fcn  Expr=sin(u(1))*tan(u(2))
  T22 : Fcn  Expr=cos(u(1))
  T23 : Fcn  Expr=sin(u(1))/cos(u(2))
  "T31 " : Fcn  Expr=cos(u(1))*tan(u(2))
  T32 : Fcn  Expr=-sin(u(1))
  T33 : Fcn  Expr=cos(u(1))/cos(u(2))
  T : Outport  OutDataType=sfix(16)  OutScaling=2^0  InitialOutput=0
  wires:
  Constant/1 -> Mux2/1
  Mux2/1 -> T/1
  theta/1 -> T23/1, T33/1, T32/1, "T31 "/1, T22/1, "T21 "/1
  T23/1 -> Mux2/6
  T22/1 -> Mux2/5
  T33/1 -> Mux2/9
  "Constant "/1 -> Mux2/2, Mux2/3
  "T21 "/1 -> Mux2/4
  "T31 "/1 -> Mux2/7
  T32/1 -> Mux2/8

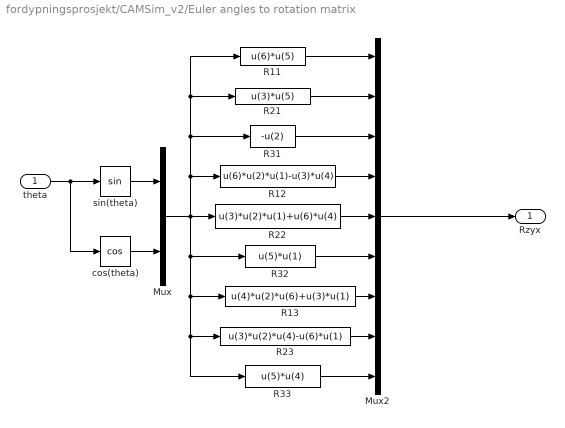
== system fordypningsprosjekt/CAMSim_v2/Euler angles to rotation matrix ==
  theta : Inport  OutDataType=sfix(16)  OutScaling=2^0
  Mux : Mux  Inputs=2
  Mux2 : Mux  Inputs=9
  R11 : Fcn  Expr=u(6)*u(5)
  R12 : Fcn  Expr=u(6)*u(2)*u(1)-u(3)*u(4)
  R13 : Fcn  Expr=u(4)*u(2)*u(6)+u(3)*u(1)
  "R21 " : Fcn  Expr=u(3)*u(5)
  R22 : Fcn  Expr=u(3)*u(2)*u(1)+u(6)*u(4)
  R23 : Fcn  Expr=u(3)*u(2)*u(4)-u(6)*u(1)
  "R31 " : Fcn  Expr=-u(2)
  R32 : Fcn  Expr=u(5)*u(1)
  R33 : Fcn  Expr=u(5)*u(4)
  cos(theta) : Trigonometry  Operator=cos
  sin(theta) : Trigonometry
  Rzyx : Outport  OutDataType=sfix(16)  OutScaling=2^0  InitialOutput=0
  wires:
  R11/1 -> Mux2/1
  Mux2/1 -> Rzyx/1
  sin(theta)/1 -> Mux/1
  cos(theta)/1 -> Mux/2
  theta/1 -> sin(theta)/1, cos(theta)/1
  Mux/1 -> R32/1, R13/1, R33/1, R23/1, R22/1, "R31 "/1, R11/1, "R21 "/1, R12/1
  R23/1 -> Mux2/8
  R13/1 -> Mux2/7
  R22/1 -> Mux2/5
  R12/1 -> Mux2/4
  "R31 "/1 -> Mux2/3
  "R21 "/1 -> Mux2/2
  R32/1 -> Mux2/6
  R33/1 -> Mux2/9

== system fordypningsprosjekt/CAMSim_v2/Euler angles to attitude transformation matrix ==
  theta : Inport  OutDataType=sfix(16)  OutScaling=2^0
  Constant : Constant  OutDataType=sfix(16)  OutScaling=2^0
  "Constant " : Constant  Value=0  OutDataType=sfix(16)  OutScaling=2^0
  Mux2 : Mux  Inputs=9
  "T21 " : Fcn  Expr=sin(u(1))*tan(u(2))
  T22 : Fcn  Expr=cos(u(1))
  T23 : Fcn  Expr=sin(u(1))/cos(u(2))
  "T31 " : Fcn  Expr=cos(u(1))*tan(u(2))
  T32 : Fcn  Expr=-sin(u(1))
  T33 : Fcn  Expr=cos(u(1))/cos(u(2))
  T : Outport  OutDataType=sfix(16)  OutScaling=2^0  InitialOutput=0
  wires:
  Constant/1 -> Mux2/1
  Mux2/1 -> T/1
  theta/1 -> T23/1, T33/1, T32/1, "T31 "/1, T22/1, "T21 "/1
  T23/1 -> Mux2/6
  T22/1 -> Mux2/5
  T33/1 -> Mux2/9
  "Constant "/1 -> Mux2/2, Mux2/3
  "T21 "/1 -> Mux2/4
  "T31 "/1 -> Mux2/7
  T32/1 -> Mux2/8

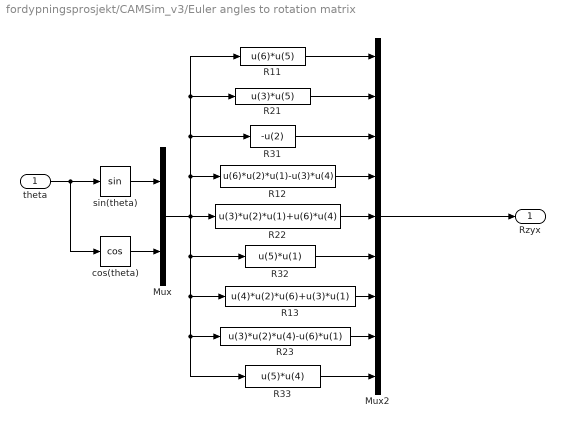
== system fordypningsprosjekt/CAMSim_v3/Euler angles to rotation matrix ==
  theta : Inport  OutDataType=sfix(16)  OutScaling=2^0
  Mux : Mux  Inputs=2
  Mux2 : Mux  Inputs=9
  R11 : Fcn  Expr=u(6)*u(5)
  R12 : Fcn  Expr=u(6)*u(2)*u(1)-u(3)*u(4)
  R13 : Fcn  Expr=u(4)*u(2)*u(6)+u(3)*u(1)
  "R21 " : Fcn  Expr=u(3)*u(5)
  R22 : Fcn  Expr=u(3)*u(2)*u(1)+u(6)*u(4)
  R23 : Fcn  Expr=u(3)*u(2)*u(4)-u(6)*u(1)
  "R31 " : Fcn  Expr=-u(2)
  R32 : Fcn  Expr=u(5)*u(1)
  R33 : Fcn  Expr=u(5)*u(4)
  cos(theta) : Trigonometry  Operator=cos
  sin(theta) : Trigonometry
  Rzyx : Outport  OutDataType=sfix(16)  OutScaling=2^0  InitialOutput=0
  wires:
  R11/1 -> Mux2/1
  Mux2/1 -> Rzyx/1
  sin(theta)/1 -> Mux/1
  cos(theta)/1 -> Mux/2
  theta/1 -> sin(theta)/1, cos(theta)/1
  Mux/1 -> R32/1, R13/1, R33/1, R23/1, R22/1, "R31 "/1, R11/1, "R21 "/1, R12/1
  R23/1 -> Mux2/8
  R13/1 -> Mux2/7
  R22/1 -> Mux2/5
  R12/1 -> Mux2/4
  "R31 "/1 -> Mux2/3
  "R21 "/1 -> Mux2/2
  R32/1 -> Mux2/6
  R33/1 -> Mux2/9

== system fordypningsprosjekt/CAMSim_v3/Euler angles to attitude transformation matrix ==
  theta : Inport  OutDataType=sfix(16)  OutScaling=2^0
  Constant : Constant  OutDataType=sfix(16)  OutScaling=2^0
  "Constant " : Constant  Value=0  OutDataType=sfix(16)  OutScaling=2^0
  Mux2 : Mux  Inputs=9
  "T21 " : Fcn  Expr=sin(u(1))*tan(u(2))
  T22 : Fcn  Expr=cos(u(1))
  T23 : Fcn  Expr=sin(u(1))/cos(u(2))
  "T31 " : Fcn  Expr=cos(u(1))*tan(u(2))
  T32 : Fcn  Expr=-sin(u(1))
  T33 : Fcn  Expr=cos(u(1))/cos(u(2))
  T : Outport  OutDataType=sfix(16)  OutScaling=2^0  InitialOutput=0
  wires:
  Constant/1 -> Mux2/1
  Mux2/1 -> T/1
  theta/1 -> T23/1, T33/1, T32/1, "T31 "/1, T22/1, "T21 "/1
  T23/1 -> Mux2/6
  T22/1 -> Mux2/5
  T33/1 -> Mux2/9
  "Constant "/1 -> Mux2/2, Mux2/3
  "T21 "/1 -> Mux2/4
  "T31 "/1 -> Mux2/7
  T32/1 -> Mux2/8

== system fordypningsprosjekt/Crusing controller/course control ==
  psi : Inport  OutDataType=sfix(16)  OutScaling=2^0
  psi_d : Inport  Port=2  OutDataType=sfix(16)  OutScaling=2^0
  r : Inport  Port=3  OutDataType=sfix(16)  OutScaling=2^0
  Gain : Gain  Gain=Kp_c  ParameterDataType=sfix(16)  ParameterScaling=2^0  OutDataType=sfix(16)  OutScaling=2^0
  Gain1 : Gain  Gain=Kd_c  ParameterDataType=sfix(16)  ParameterScaling=2^0  OutDataType=sfix(16)  OutScaling=2^0
  Gain2 : Gain  Gain=5  ParameterDataType=sfix(16)  ParameterScaling=2^0  OutDataType=sfix(16)  OutScaling=2^0
  Gain3 : Gain  Gain=0.1  ParameterDataType=sfix(16)  ParameterScaling=2^0  OutDataType=sfix(16)  OutScaling=2^0
  Sum : Sum  Inputs=|+-  OutDataType=sfix(16)  OutScaling=2^0
  Sum1 : Sum  Inputs=|-+  OutDataType=sfix(16)  OutScaling=2^0
  tau_2 : Outport  OutDataType=sfix(16)  OutScaling=2^0
  tau_6 : Outport  Port=2  OutDataType=sfix(16)  OutScaling=2^0
  wires:
  Sum/1 -> Gain3/1, Gain2/1
  r/1 -> Gain1/1
  Gain/1 -> Sum/1
  psi_d/1 -> Sum1/2
  psi/1 -> Sum1/1
  Gain1/1 -> Sum/2
  Sum1/1 -> Gain/1
  Gain2/1 -> tau_6/1
  Gain3/1 -> tau_2/1

== system fordypningsprosjekt/Crusing controller/depth ==
  D : Inport  OutDataType=sfix(16)  OutScaling=2^0
  D_d : Inport  Port=2  OutDataType=sfix(16)  OutScaling=2^0
  q : Inport  Port=3  OutDataType=sfix(16)  OutScaling=2^0
  theta : Inport  Port=4  OutDataType=sfix(16)  OutScaling=2^0
  Gain : Gain  Gain=Kp_d  ParameterDataType=sfix(16)  ParameterScaling=2^0  OutDataType=sfix(16)  OutScaling=2^0
  Gain1 : Gain  Gain=Kd_d  ParameterDataType=sfix(16)  ParameterScaling=2^0  OutDataType=sfix(16)  OutScaling=2^0
  Gain2 : Gain  Gain=-2  ParameterDataType=sfix(16)  ParameterScaling=2^0  OutDataType=sfix(16)  OutScaling=2^0
  Gain3 : Gain  Gain=Kp2_d  ParameterDataType=sfix(16)  ParameterScaling=2^0  OutDataType=sfix(16)  OutScaling=2^0
  Sum : Sum  Inputs=+--  OutDataType=sfix(16)  OutScaling=2^0
  Sum1 : Sum  Inputs=|-+  OutDataType=sfix(16)  OutScaling=2^0
  tau_3 : Outport  OutDataType=sfix(16)  OutScaling=2^0
  tau_5 : Outport  Port=2  OutDataType=sfix(16)  OutScaling=2^0
  wires:
  Gain3/1 -> Sum/3
  theta/1 -> Gain3/1
  Sum1/1 -> Gain/1
  Gain1/1 -> Sum/2
  D/1 -> Sum1/1
  D_d/1 -> Sum1/2
  Gain/1 -> Sum/1
  q/1 -> Gain1/1
  Sum/1 -> Gain2/1, tau_3/1
  Gain2/1 -> tau_5/1

== system fordypningsprosjekt/Crusing controller/speed ==
  u : Inport  OutDataType=sfix(16)  OutScaling=2^0
  u_d : Inport  Port=2  OutDataType=sfix(16)  OutScaling=2^0
  Gain : Gain  Gain=Ki_u  ParameterDataType=sfix(16)  ParameterScaling=2^0  OutDataType=sfix(16)  OutScaling=2^0
  Gain1 : Gain  Gain=Kp_u  ParameterDataType=sfix(16)  ParameterScaling=2^0  OutDataType=sfix(16)  OutScaling=2^0
  Integrator : Integrator
  Sum : Sum  Inputs=|--  OutDataType=sfix(16)  OutScaling=2^0
  Sum1 : Sum  Inputs=|+-  OutDataType=sfix(16)  OutScaling=2^0
  Out1 : Outport  OutDataType=sfix(16)  OutScaling=2^0
  wires:
  Gain1/1 -> Sum/2
  Gain/1 -> Integrator/1
  Integrator/1 -> Sum/1
  Sum1/1 -> Gain1/1, Gain/1
  u_d/1 -> Sum1/2
  u/1 -> Sum1/1
  Sum/1 -> Out1/1

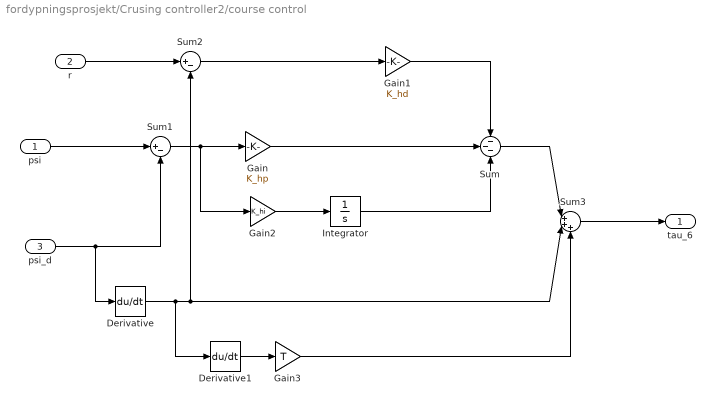
== system fordypningsprosjekt/Crusing controller2/course control ==
  psi : Inport  OutDataType=sfix(16)  OutScaling=2^0
  r : Inport  Port=2  OutDataType=sfix(16)  OutScaling=2^0
  psi_d : Inport  Port=3  OutDataType=sfix(16)  OutScaling=2^0
  Derivative : Derivative
  Derivative1 : Derivative
  Gain : Gain  Gain=K_hp  ParameterDataType=sfix(16)  ParameterScaling=2^0  OutDataType=sfix(16)  OutScaling=2^0
  Gain1 : Gain  Gain=K_hd  ParameterDataType=sfix(16)  ParameterScaling=2^0  OutDataType=sfix(16)  OutScaling=2^0
  Gain2 : Gain  Gain=K_hi  ParameterDataType=sfix(16)  ParameterScaling=2^0  OutDataType=sfix(16)  OutScaling=2^0
  Gain3 : Gain  Gain=T  ParameterDataType=sfix(16)  ParameterScaling=2^0  OutDataType=sfix(16)  OutScaling=2^0
  Integrator : Integrator
  Sum : Sum  Inputs=---  OutDataType=sfix(16)  OutScaling=2^0
  Sum1 : Sum  Inputs=|+-  OutDataType=sfix(16)  OutScaling=2^0
  Sum2 : Sum  Inputs=|+-  OutDataType=sfix(16)  OutScaling=2^0
  Sum3 : Sum  Inputs=|+++  OutDataType=sfix(16)  OutScaling=2^0
  tau_6 : Outport  OutDataType=sfix(16)  OutScaling=2^0
  wires:
  Gain3/1 -> Sum3/3
  Derivative1/1 -> Gain3/1
  Derivative/1 -> Derivative1/1, Sum3/2, Sum2/2
  Sum2/1 -> Gain1/1
  r/1 -> Sum2/1
  Sum1/1 -> Gain/1, Gain2/1
  psi/1 -> Sum1/1
  psi_d/1 -> Derivative/1, Sum1/2
  Gain2/1 -> Integrator/1
  Gain/1 -> Sum/2
  Integrator/1 -> Sum/3
  Gain1/1 -> Sum/1
  Sum/1 -> Sum3/1
  Sum3/1 -> tau_6/1

== system fordypningsprosjekt/Crusing controller2/depth ==
  D : Inport  OutDataType=sfix(16)  OutScaling=2^0
  D_d : Inport  Port=2  OutDataType=sfix(16)  OutScaling=2^0
  theta : Inport  Port=3  OutDataType=sfix(16)  OutScaling=2^0
  q : Inport  Port=4  OutDataType=sfix(16)  OutScaling=2^0
  Gain : Gain  Gain=K_dp  ParameterDataType=sfix(16)  ParameterScaling=2^0  OutDataType=sfix(16)  OutScaling=2^0
  Gain2 : Gain  Gain=K_dd  ParameterDataType=sfix(16)  ParameterScaling=2^0  OutDataType=sfix(16)  OutScaling=2^0
  Gain3 : Gain  Gain=K_dd  ParameterDataType=sfix(16)  ParameterScaling=2^0  OutDataType=sfix(16)  OutScaling=2^0
  Sum : Sum  Inputs=-++  OutDataType=sfix(16)  OutScaling=2^0
  Sum1 : Sum  Inputs=|-+  OutDataType=sfix(16)  OutScaling=2^0
  tau_5 : Outport  OutDataType=sfix(16)  OutScaling=2^0
  wires:
  Gain3/1 -> Sum/3
  Gain2/1 -> Sum/2
  q/1 -> Gain3/1
  Sum/1 -> tau_5/1
  Gain/1 -> Sum/1
  D_d/1 -> Sum1/2
  D/1 -> Sum1/1
  Sum1/1 -> Gain/1
  theta/1 -> Gain2/1

== system fordypningsprosjekt/Crusing controller2/speed ==
  u : Inport  OutDataType=sfix(16)  OutScaling=2^0
  u_d : Inport  Port=2  OutDataType=sfix(16)  OutScaling=2^0
  Gain : Gain  Gain=Ki_u  ParameterDataType=sfix(16)  ParameterScaling=2^0  OutDataType=sfix(16)  OutScaling=2^0
  Gain1 : Gain  Gain=Kp_u  ParameterDataType=sfix(16)  ParameterScaling=2^0  OutDataType=sfix(16)  OutScaling=2^0
  Integrator : Integrator
  Sum : Sum  Inputs=|--  OutDataType=sfix(16)  OutScaling=2^0
  Sum1 : Sum  Inputs=|+-  OutDataType=sfix(16)  OutScaling=2^0
  Out1 : Outport  OutDataType=sfix(16)  OutScaling=2^0
  wires:
  Sum/1 -> Out1/1
  u/1 -> Sum1/1
  u_d/1 -> Sum1/2
  Sum1/1 -> Gain/1, Gain1/1
  Integrator/1 -> Sum/1
  Gain/1 -> Integrator/1
  Gain1/1 -> Sum/2
